simulink model "tutorial37_triggered"  (R2025a)
settings: Solver=VariableStepAuto  StartTime=0.0  StopTime=10.0  RelTol=1e-3
settings Model: Creator=xing2  LastModifiedBy=xing2

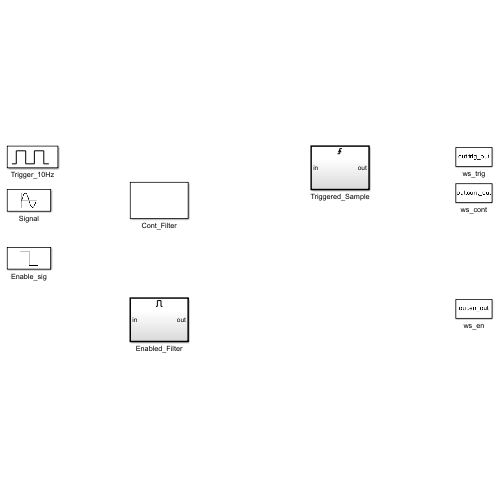
[thumbnail: Simulink's stored preview of the top-level diagram]
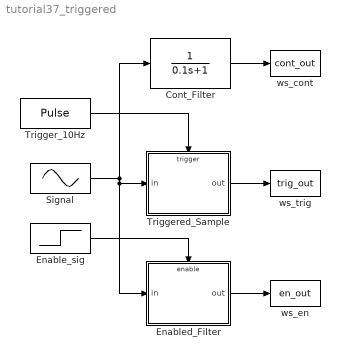
== system tutorial37_triggered ==
  Cont_Filter : TransferFcn  Denominator=[0.1 1]
  Enable_sig : Step  Time=2  Before=1  After=0  SampleTime=0
  Enabled_Filter : Subsystem  TreatAsAtomicUnit=on
  Signal : Sin  Frequency=2  SampleTime=0
  Trigger_10Hz : DiscretePulseGenerator  PulseType=Time based  Period=0.1  PulseWidth=50
  Triggered_Sample : Subsystem  TreatAsAtomicUnit=on
  ws_cont : ToWorkspace  VariableName=cont_out  SaveFormat=Timeseries  SampleTime=-1
  ws_en : ToWorkspace  VariableName=en_out  SaveFormat=Timeseries  SampleTime=-1
  ws_trig : ToWorkspace  VariableName=trig_out  SaveFormat=Timeseries  SampleTime=-1
  wires:
  Triggered_Sample/1(out) -> ws_trig/1
  Signal/1 -> Enabled_Filter/1(in), Triggered_Sample/1(in), Cont_Filter/1
  Trigger_10Hz/1 -> Triggered_Sample/Trigger
  Enable_sig/1 -> Enabled_Filter/Enable
  Cont_Filter/1 -> ws_cont/1
  Enabled_Filter/1(out) -> ws_en/1

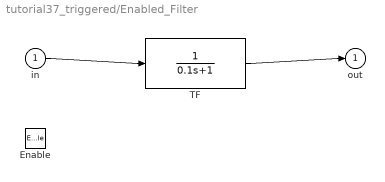
== system tutorial37_triggered/Enabled_Filter ==
  in : Inport
  Enable : EnablePort
  TF : TransferFcn  Denominator=[0.1 1]
  out : Outport
  wires:
  in/1 -> TF/1
  TF/1 -> out/1

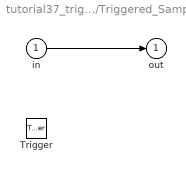
== system tutorial37_triggered/Triggered_Sample ==
  in : Inport
  Trigger : TriggerPort  VariantControl=(inherit)  PortDimensions=1
  out : Outport
  wires:
  in/1 -> out/1
